simulink model "xts_system"  (R2026a)
settings: Solver=ode45  MaxStep=1e-2  AbsTol=1e-3
PreLoadFcn:
  | xts_PARAM
undefined symbols (not defined in the file or in its folder): sigbuilder_block, station_data, X, xts_rail_color, xts_rail_extr, xts_track_seg, Y, Z
libraries: sm_lib x28, xts_movers_lib x4, Multibody_Parts_Lib x4, nesl_utility x1
CloseFcn:
  | try,close(h1_xts_system),end
  | clear h1_xts_system
  | try,close(h2_xts_system),end
  | clear h2_xts_system
  | try,close(h3_xts_system),end
  | clear h3_xts_system
  | 
  | clear simlog_xts_system
  | clear logsout_xts_system
Description:
  | Linear Transport System
  | 
  | Copyright 2017-2026 The MathWorks, Inc.
settings Model: Creator=smiller  LastModifiedBy=smiller
settings DataIOCC: SignalLoggingName=logsout_xts_system
settings DebuggingCC: PregeneratedLibrarySubsystemCodeDiagnostic=none
settings SimscapeCC: SimscapeNormalizeSystem=off  SimscapeNominalValues="[{\"value\":\"1\",\"unit\":\"A\"},{\"value\":\"1\",\"unit\":\"bar\"},{\"value\":\"1\",\"unit\":\"cm^2\"},{\"value\":\"1\",\"unit\":\"cm^3/s\"},{\"value\":\"1\",\"unit\":\"kJ/kg\"},{\"value\":\"1\",\"unit\":\"kW\"},{\"value\":\"1\",\"unit\":\"l\"},{\"value\":\"1\",\"unit\":\"N\"},{\"value\":\"1\",\"unit\":\"N*m\"},{\"value\":\"1\",\"unit\":\"V\"}]"  SimscapeLogSimulationStatistics=on  SimscapeLogName=simlog_xts_system
settings DiagnosticsConfigSet: SimMechanicsUnconnectedFramePorts=none
settings ExplorerConfigSet: InternalSimMechanicsExplorerSettings="<ExplorerConfiguration><canonicalview>default</canonicalview><AnimationSetting><BasePlaybackSpeed>1.0</BasePlaybackSpeed><PlaybackSpeedFactor>1.0</PlaybackSpeedFactor></AnimationSetting><TilePanel><TileInfo><Tiles Columns=\"1\" Count=\"2\" Rows=\"2\"><Column Left=\"2\" Weight=\"1\"/><Column Left=\"429\"/><Row Top=\"2\" Weight=\"0.5743\"/><Row Top=\"165\" Weight=\"0.4257\"/><Row Top=\"287\"/><Tile Height=\"1\" Width=\"1\" X=\"0\" Y=\"0\"/><Tile Height=\"1\" Width=\"1\" X=\"0\" Y=\"1\"/></Tiles></TileInfo><SceneInfo><SceneViewer><BGColor><R>1</R><G>1</G><B>1</B></BGColor><Camera><DoPerspective>off</DoPerspective><Position><X>0.85235026960784244</X><Y>-0.74235025649298092</Y><Z>0.57735026635840536</Z></Position><Center><X>0.27500000041821659</X><Y>-0.16499998730335524</Y><Z>-2.831220369259313e-09</Z></Center><Up><X>-0.40824829046386307</X><Y>0.40824829046386307</Y><Z>0.81649658092772615</Z></Up><ViewLimDist>1</ViewLimDist><YLim>0.29785614758729934</YLim><XLim>0.80846668630838392</XLim></Camera></SceneViewer><SceneViewer><BGColor><R>1</R><G>1</G><B>1</B></BGColor><Camera><DoPerspective>on</DoPerspective><Position><X>-0.0044513318879480434</X><Y>-7.988545794836407e-05</Y><Z>0.039999999999999994</Z></Position><Center><X>0.99519221354671583</X><Y>0.026618093319754715</Y><Z>0.03999999999999955</Z></Center><Up><X>2.2204460492503131e-16</X><Y>0</Y><Z>0.99999999999999978</Z></Up><ViewLimDist>1</ViewLimDist><YLim>0.46630765815499858</YLim><XLim>1.7249256735291099</XLim></Camera></SceneViewer></SceneInfo></TilePanel><MechEditorPanel><Cameras><Camera><Id>Camera1</Id><Value><Name>Mover1</Name><NativeCamera><PositionTrackingFeature>Conveyor_1.Mover_1.Mover.Transform_Camera_1.F</PositionTrackingFeature><CenterTrackingFeature>Conveyor_1.Mover_1.Mover.Transform_Camera_1.F</CenterTrackingFeature><UpVectorTrackingFeature>Conveyor_1.Mover_1.Mover.Transform_Camera_1.F</UpVectorTrackingFeature><CenterTrackingOrigin>off</CenterTrackingOrigin><CenterTrackingDirection>-Z</CenterTrackingDirection><UpVectorTrackingDirection>-Y</UpVectorTrackingDirection></NativeCamera></Value></Camera></Cameras><GfxPanelCameraMap><MapElement CameraMLId=\"Camera1\" GfxPanelIndex=\"1\"/></GfxPanelCameraMap><VideoCreator><PlaybackSpeedRatio>1.0</PlaybackSpeedRatio><FrameRate>30</FrameRate><VideoFormat>Motion JPEG AVI</VideoFormat><FrameSize>auto</FrameSize></VideoCreator></MechEditorPanel></ExplorerConfiguration>"

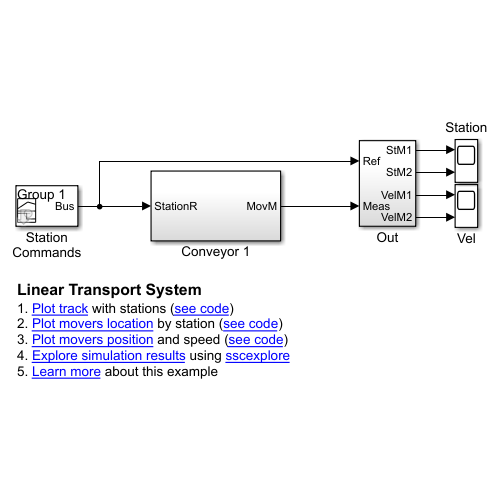
[thumbnail: Simulink's stored preview of the top-level diagram]
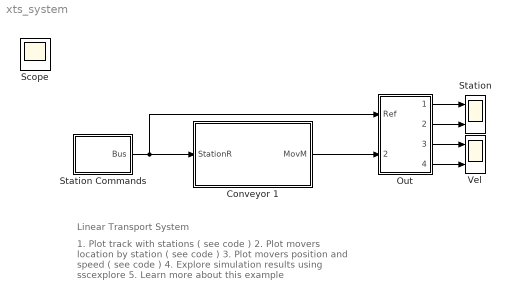
== system xts_system ==
  note: Linear Transport System
  note: 1. Plot track with stations ( see code )
      | 2. Plot movers location by station ( see code )
      | 3. Plot movers position and speed ( see code )
      | 4. Explore simulation results using sscexplore
      | 5. Learn more about this example
  Conveyor 1 : Subsystem  Tag=PublishSubsystem
  Out : Subsystem
  Station : Scope  NumInputPorts=2
      settings: ActiveDisplayYMinimum=-1.5  ActiveDisplayYMaximum=13.5  DataLoggingVariableName=ScopeData3
  Station Commands : Subsystem  Tag=STV Subsys  LoadFcn=sigbuilder_block('load');  StartFcn=sigbuilder_block('start');  StopFcn=sigbuilder_block('stop');  ClipboardFcn=sigbuilder_block('clipboard');  mask(Sigbuilder block){tuvar=[0:10]}
      mask help: Simulink:masks:SigbuilderBlock_MD
      mask init:
      | if ~strcmp(get_param(bdroot(gcbh),'SimulationStatus'),'stopped') tuvar = sigbuilder_block('maskInit'); end
      settings: CopyFcn=sigbuilder_block('copy');  DeleteFcn=sigbuilder_block('delete');  ModelCloseFcn=sigbuilder_block('modelClose');  PreSaveFcn=sigbuilder_block('preSave');  PauseFcn=sigbuilder_block('pause');  ContinueFcn=sigbuilder_block('continue');  NameChangeFcn=sigbuilder_block('namechange');  OpenFcn=sigbuilder_block('open',[437.6 199.2 550.4 400 ]);  CloseFcn=sigbuilder_block('close');
      mask Display: plot(0, 0, 100, 100,[2, 2, 32, 32, 2], [68, 8, 8, 68, 68],[32, 2], [38, 38], [32, 19, 2],[53, 60, 44], [32, 17, 17, 2],[16, 16, 31, 31]);txt = getActiveGroup(gcbh);text(2, 100, txt,'verticalAlignment', 'top');
  Vel : Scope  NumInputPorts=2
      settings: ActiveDisplayYMinimum=-0.12686  ActiveDisplayYMaximum=1.14176
  Scope : Scope
      settings: ActiveDisplayYMinimum=-6.25  ActiveDisplayYMaximum=56.25
  wires:
  Station Commands/1(Bus) -> Out/1(Ref), Conveyor 1/1(StationR)
  Conveyor 1/1(MovM) -> Out/2(Meas)
  Out/1(StM1) -> Station/1
  Out/2(StM2) -> Station/2
  Out/3(VelM1) -> Vel/1
  Out/4(VelM2) -> Vel/2

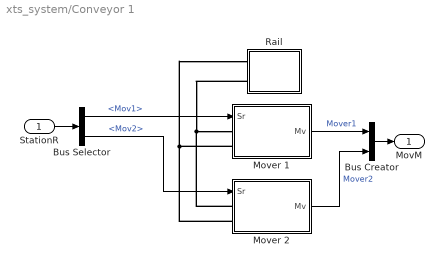
== system xts_system/Conveyor 1 ==
  StationR : Inport
  Bus Creator : BusCreator  Inputs=2
  Bus Selector : BusSelector  OutputSignals=Mov1,Mov2
  Mover 1 : Subsystem  Tag=PublishSubsystem
  Mover 2 : Subsystem
  Rail : Subsystem
  MovM : Outport  VectorParamsAs1DForOutWhenUnconnected=off
  wires:
  StationR/1 -> Bus Selector/1
  Bus Selector/1 -> Mover 1/1(Sr)  "<Mov1>"
  Bus Selector/2 -> Mover 2/1(Sr)  "<Mov2>"
  Mover 1/1(Mv) -> Bus Creator/1  "Mover1"
  Mover 2/1(Mv) -> Bus Creator/2  "Mover2"
  Bus Creator/1 -> MovM/1
  connections:
  Mover 1/LConn2 -- Mover 2/LConn2 -- Rail/RConn1
  Rail/RConn2 -- Mover 2/LConn1 -- Mover 1/LConn1

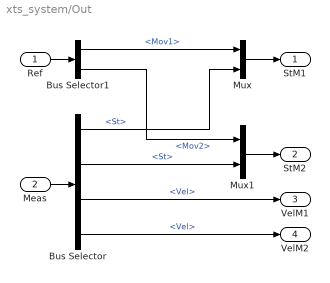
== system xts_system/Out ==
  Ref : Inport
  Meas : Inport  Port=2
  Bus Selector : BusSelector  OutputSignals=Mover1.St,Mover2.St,Mover1.Vel,Mover2.Vel
  Bus Selector1 : BusSelector  OutputSignals=Mov1,Mov2
  Mux : Mux  Inputs=2
  Mux1 : Mux  Inputs=2
  StM1 : Outport  VectorParamsAs1DForOutWhenUnconnected=off
  StM2 : Outport  Port=2  VectorParamsAs1DForOutWhenUnconnected=off
  VelM1 : Outport  Port=3  VectorParamsAs1DForOutWhenUnconnected=off
  VelM2 : Outport  Port=4  VectorParamsAs1DForOutWhenUnconnected=off
  wires:
  Bus Selector/1 -> Mux/2  "<St>"
  Mux/1 -> StM1/1
  Bus Selector1/2 -> Mux1/1  "<Mov2>"
  Mux1/1 -> StM2/1
  Bus Selector/4 -> VelM2/1  "<Vel>"
  Bus Selector/3 -> VelM1/1  "<Vel>"
  Bus Selector1/1 -> Mux/1  "<Mov1>"
  Meas/1 -> Bus Selector/1
  Bus Selector/2 -> Mux1/2  "<St>"
  Ref/1 -> Bus Selector1/1

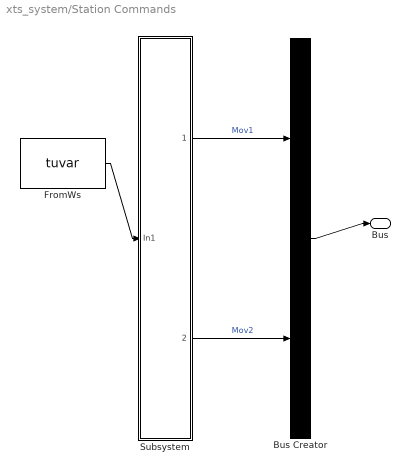
== system xts_system/Station Commands ==
  Bus Creator : BusCreator  Tag=Bus Creator  Inputs=2
  FromWs : FromWorkspace  Tag=STV FromWs  VariableName=tuvar
      SigBuilderData=|
      | common.afterFinalStr = 'Extrapolate'
      | common.sampleTime = 0
      | dataSet.timeRange = [0 10]
      | dataSet.name = 'Group 1'
      | sbobj.Groups.Name = 'Group 1'
      | sbobj.Groups.Signals(1).Name = 'Mov1'
      | sbobj.Groups.Signals(1).XData = [0 1.36 1.36 4 4 6 6 10]
      | sbobj.Groups.Signals(1).YData = [1 1 3 3 5 5 1 1]
      | sbobj.Groups.Signals(2).Name = 'Mov2'
      | sbobj.Groups.Signals(2).XData = [0 2.8 2.8 5 5 7.46 7.46 10]
      | sbobj.Groups.Signals(2).YData = [1 1 2 2 4 4 6 6]
  Subsystem : Subsystem
  Bus : Outport  VectorParamsAs1DForOutWhenUnconnected=off
  wires:
  FromWs/1 -> Subsystem/1(In1)
  Subsystem/1(Mov1) -> Bus Creator/1  "Mov1"
  Subsystem/2(Mov2) -> Bus Creator/2  "Mov2"
  Bus Creator/1 -> Bus/1

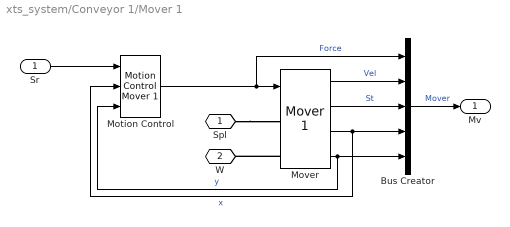
== system xts_system/Conveyor 1/Mover 1 ==
  Sr : Inport
  Bus Creator : BusCreator  Inputs=5
  Motion Control : xts_movers_lib/Motion Control Mover 1  dead_zone=xts_ctrl_dead_zone  max_force=xts_ctrl_max_force  err_gain_on_off=xts_ctrl_on_off_gain
  Mover : xts_movers_lib/Mover 1  Tag=PublishSubsystem  vis_popup=Native  visc_friction=xts_rail_visc_frict  init_pos_xy=[0 0]  station_data_o=station_o  station_data_x=station_x  station_data_y=station_y
  Spl : PMIOPort  Side=Left
  W : PMIOPort  Port=2  Side=Left
  Mv : Outport  VectorParamsAs1DForOutWhenUnconnected=off
  wires:
  Sr/1 -> Motion Control/1
  Mover/2 -> Bus Creator/3  "St"
  Mover/1 -> Bus Creator/2  "Vel"
  Motion Control/1 -> Bus Creator/1, Mover/1  "Force"
  Mover/3 -> Bus Creator/4, Motion Control/2  "x"
  Mover/4 -> Bus Creator/5, Motion Control/3  "y"
  Bus Creator/1 -> Mv/1  "Mover"
  connections:
  Mover/LConn2 -- W/RConn1
  Spl/RConn1 -- Mover/LConn1

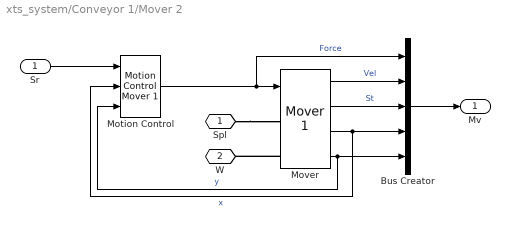
== system xts_system/Conveyor 1/Mover 2 ==
  Sr : Inport
  Bus Creator : BusCreator  Inputs=5
  Motion Control : xts_movers_lib/Motion Control Mover 1  dead_zone=xts_ctrl_dead_zone  max_force=xts_ctrl_max_force  err_gain_on_off=xts_ctrl_on_off_gain
  Mover : xts_movers_lib/Mover 1  vis_popup=Native  visc_friction=xts_rail_visc_frict  init_pos_xy=[0.5 0]  station_data_o=station_o  station_data_x=station_x  station_data_y=station_y
  Spl : PMIOPort  Side=Left
  W : PMIOPort  Port=2  Side=Left
  Mv : Outport  VectorParamsAs1DForOutWhenUnconnected=off
  wires:
  Bus Creator/1 -> Mv/1
  Mover/4 -> Motion Control/3, Bus Creator/5  "y"
  Mover/3 -> Motion Control/2, Bus Creator/4  "x"
  Motion Control/1 -> Mover/1, Bus Creator/1  "Force"
  Mover/1 -> Bus Creator/2  "Vel"
  Mover/2 -> Bus Creator/3  "St"
  Sr/1 -> Motion Control/1
  connections:
  Spl/RConn1 -- Mover/LConn1
  Mover/LConn2 -- W/RConn1

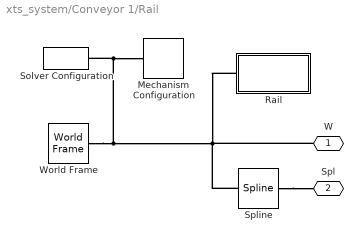
== system xts_system/Conveyor 1/Rail ==
  Mechanism Configuration : sm_lib/Utilities/Mechanism Configuration  UniformGravity=Constant  GravityVector=[0 -9.80665 0]*0  GravityVectorUnits=m/s^2  LinearizationDelta=0.001  JointModeTransitionNonlinearIterations=2
  Rail : Subsystem  Tag=PublishSubsystem  mask{rail_xc=xts_rail_extr, rail_seg=xts_track_seg, rail_color=xts_rail_color}
      mask prompts: rail_xc "Rail Cross-Section in x-y (m)"; rail_seg "Track Segments (len/rad, angle)"; rail_color "Rail Color (RGB)"
  Solver Configuration : nesl_utility/Solver Configuration  PhysicalDomain=network_engine_domain  SubClassName=solver  LeftPortType=input  RightPortType=generic  Tones=[]  Harmonics=[]  SimulateNoise=off  Profile=off  UseLocalSampling=off  EnableSwitchedLinearOptims=on  FrequencyDomain=off  UseCCode=off  RelTol=0.001  AbsTol=1e-06  MinStep=1e-09  ToWorkspace=off  RevertToSquareIcSolve=off  NumHomotopyIterations=100  PhasorMode=off  PhasorModeNumHarmonics=1  ConsistencySolver=NEWTON_FTOL  CanonicalOrdering=UNORDERED  OptimizeIntermediates=UNOPTIMIZED  IndexReductionMethod=DerivativeReplacement  DoDC=off  ResidualTolerance=1e-09  ConsistencyTolSource=GLOBAL  ConsistencyAbsTol=0.001  ConsistencyRelTol=0.001  ConsistencyTolFactor=0.001  UseLocalSolver=off  LocalSolverChoice=NE_BACKWARD_EULER_ADVANCER  ResolveIndetEquations=on  FunctionEvalNumThread=1  LocalSolverSampleTime=0.001  DoFixedCost=off  MaxNonlinIter=3  MaxModeIter=2  ComputeImpulses=off  ImpulseIterations=2  LinearAlgebra=Sparse  LinearAlgebraNumThread=0  EquationFormulation=NE_TIME_EF  DelaysMemoryBudget=1024  AutomaticFiltering=on  FilteringTimeConstant=0.001  PartitionStorageMethod=AS_NEEDED  PartitionMemoryBudget=1024  PartitionMethod=FAST  MultibodyUseLocalSolver=off  MultibodyLocalSolverChoice=ODE1  MultibodyLocalSolverSampleTime=0.001
  Spline : sm_lib/Curves and Surfaces/Spline  DataPoints=rail_spline  DataPointsUnits=m  EndConditionType=Closed  GraphicType=FromGeometry  MarkerShape=Sphere  MarkerSize=10  GraphicVisPropType=SimpleVisualProperties  GraphicDiffuseColor=[0 0 0]  GraphicOpacity=1.0  GraphicSpecularColor=[0.5 0.5 0.5 1.0]  GraphicAmbientColor=[0.15 0.15 0.15 1.0]  GraphicEmissiveColor=[0.0 0.0 0.0 1.0]  GraphicShininess=75
  World Frame : sm_lib/Frames and Transforms/World Frame
  W : PMIOPort  Side=Right
  Spl : PMIOPort  Port=2  Side=Right
  connections:
  Spline/RConn1 -- Spl/RConn1
  Solver Configuration/RConn1 -- W/RConn1 -- Spline/LConn1 -- Rail/LConn1 -- World Frame/RConn1 -- Mechanism Configuration/RConn1

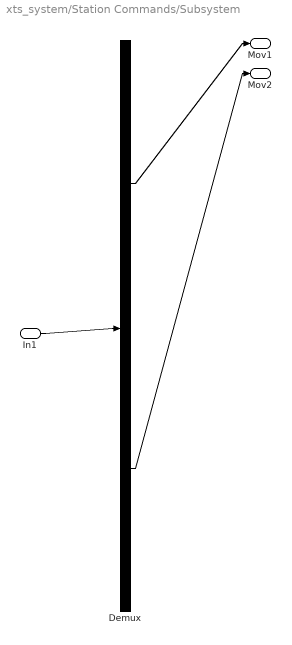
== system xts_system/Station Commands/Subsystem ==
  In1 : Inport
  Demux : Demux  Tag=STV Demux  Outputs=2
      settings: DisplayOption=none
  Mov1 : Outport  Tag=STV Outport  VectorParamsAs1DForOutWhenUnconnected=off
  Mov2 : Outport  Tag=STV Outport  Port=2  VectorParamsAs1DForOutWhenUnconnected=off
  wires:
  Demux/1 -> Mov1/1
  Demux/2 -> Mov2/1
  In1/1 -> Demux/1

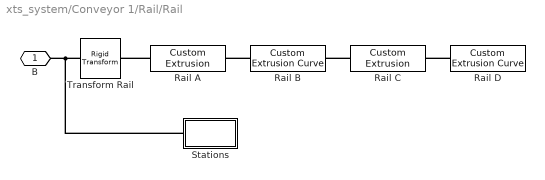
== system xts_system/Conveyor 1/Rail/Rail ==
  Rail A : Multibody_Parts_Lib/Extrusions/Custom Extrusion  extr_xsec=rail_xc  extr_len=rail_seg(1,1)  extr_rho=7000  extr_color=rail_color  extr_opc=1
      settings: SourceProductName=Simscape Multibody Parts Library
  Rail B : Multibody_Parts_Lib/Extrusions/Custom Extrusion Curve  extr_xsec=rail_xc  arc_rad=rail_seg(2,1)  arc_angle=rail_seg(2,2)  popup_arcdir=Y  extr_rho=7000  extr_color=rail_color  extr_opc=1
      settings: SourceProductName=Simscape Multibody Parts Library
  Rail C : Multibody_Parts_Lib/Extrusions/Custom Extrusion  extr_xsec=rail_xc  extr_len=rail_seg(3,1)  extr_rho=7000  extr_color=rail_color  extr_opc=1
      settings: SourceProductName=Simscape Multibody Parts Library
  Rail D : Multibody_Parts_Lib/Extrusions/Custom Extrusion Curve  extr_xsec=rail_xc  arc_rad=rail_seg(4,1)  arc_angle=rail_seg(4,2)  popup_arcdir=Y  extr_rho=7000  extr_color=rail_color  extr_opc=1
      settings: SourceProductName=Simscape Multibody Parts Library
  Stations : Subsystem
  Transform Rail : sm_lib/Frames and Transforms/Rigid Transform  RotationMethod=StandardAxis  FollAlignAxisA=+Z  BaseAlignAxisA=+X  FollAlignAxisB=+X  BaseAlignAxisB=-Y  RotationStandardAxis=+X  RotationAngle=-90  RotationAngleUnits=deg  RotationArbitraryAxis=[0 0 1]  RotationSequenceAxes=FollowerAxes  RotationSequence=XYX  RotationSequenceAngles=[0 0 0]  RotationSequenceAnglesUnits=deg  RotationMatrix=[1 0 0; 0 1 0; 0 0 1]  Quaternion=[1 0 0 0]  TranslationMethod=None  TranslationCartesianOffset=[0 0 0]  TranslationCartesianOffsetUnits=m  TranslationStandardAxis=+Z  TranslationStandardOffset=0  TranslationStandardOffsetUnits=m  TranslationROffset=0  TranslationROffsetUnits=m  TranslationThetaOffset=0  TranslationThetaOffsetUnits=deg  TranslationZOffset=0  TranslationZOffsetUnits=m
  B : PMIOPort  Side=Left
  connections:
  Stations/LConn1 -- Transform Rail/LConn1 -- B/RConn1
  Rail B/LConn1 -- Rail A/RConn1
  Rail D/LConn1 -- Rail C/RConn1
  Rail C/LConn1 -- Rail B/RConn1
  Rail A/LConn1 -- Transform Rail/RConn1

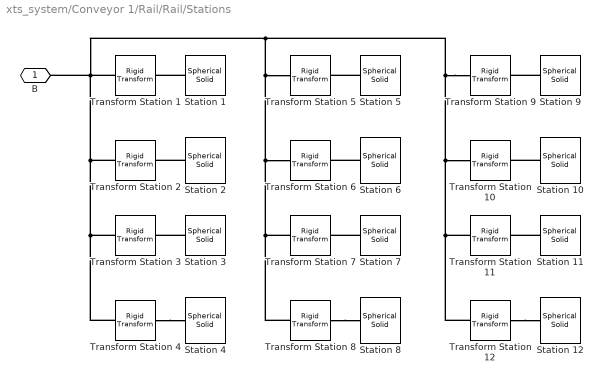
== system xts_system/Conveyor 1/Rail/Rail/Stations ==
  Station {1..12} (12 alike) : sm_lib/Body Elements/Spherical Solid  SphereRadius=0.05  SphereRadiusUnits=m  ExportEntireGeometry=off  InertiaType=CalculateFromGeometry  BasedOnType=Density  Density=1000  DensityUnits=kg/m^3  Mass=1  MassUnits=kg  CenterOfMass=[0 0 0]  CenterOfMassUnits=m  MomentsOfInertia=[1 1 1]  MomentsOfInertiaUnits=kg*m^2  ProductsOfInertia=[1 1 1]  ProductsOfInertiaUnits=kg*m^2  GraphicType=FromGeometry  MarkerShape=Sphere  MarkerSize=10  GraphicVisPropType=SimpleVisualProperties  GraphicDiffuseColor=[1.0 0.6 0.4]  GraphicOpacity=0.3  GraphicSpecularColor=[0.5 0.5 0.5 1.0]  GraphicAmbientColor=[0.15 0.15 0.15 1.0]  GraphicEmissiveColor=[0.0 0.0 0.0 1.0]  GraphicShininess=75  DoExposeReferenceFrame=on  SerializedFrames=<Frames/>
  Transform Station 1 : sm_lib/Frames and Transforms/Rigid Transform  RotationMethod=None  FollAlignAxisA=+X  BaseAlignAxisA=+Y  FollAlignAxisB=+Y  BaseAlignAxisB=+Z  RotationStandardAxis=+X  RotationAngle=0  RotationAngleUnits=deg  RotationArbitraryAxis=[0 0 1]  RotationSequenceAxes=FollowerAxes  RotationSequence=XYX  RotationSequenceAngles=[0 0 0]  RotationSequenceAnglesUnits=deg  RotationMatrix=[1 0 0; 0 1 0; 0 0 1]  Quaternion=[1 0 0 0]  TranslationMethod=Cartesian  TranslationCartesianOffset=[station_data(1,2) station_data(1,3) 0]  TranslationCartesianOffsetUnits=m  TranslationStandardAxis=+Z  TranslationStandardOffset=0  TranslationStandardOffsetUnits=m  TranslationROffset=0  TranslationROffsetUnits=m  TranslationThetaOffset=0  TranslationThetaOffsetUnits=deg  TranslationZOffset=0  TranslationZOffsetUnits=m
  Transform Station 10 : sm_lib/Frames and Transforms/Rigid Transform  RotationMethod=None  FollAlignAxisA=+X  BaseAlignAxisA=+Y  FollAlignAxisB=+Y  BaseAlignAxisB=+Z  RotationStandardAxis=+X  RotationAngle=0  RotationAngleUnits=deg  RotationArbitraryAxis=[0 0 1]  RotationSequenceAxes=FollowerAxes  RotationSequence=XYX  RotationSequenceAngles=[0 0 0]  RotationSequenceAnglesUnits=deg  RotationMatrix=[1 0 0; 0 1 0; 0 0 1]  Quaternion=[1 0 0 0]  TranslationMethod=Cartesian  TranslationCartesianOffset=[station_data(10,2) station_data(10,3) 0]  TranslationCartesianOffsetUnits=m  TranslationStandardAxis=+Z  TranslationStandardOffset=0  TranslationStandardOffsetUnits=m  TranslationROffset=0  TranslationROffsetUnits=m  TranslationThetaOffset=0  TranslationThetaOffsetUnits=deg  TranslationZOffset=0  TranslationZOffsetUnits=m
  Transform Station 11 : sm_lib/Frames and Transforms/Rigid Transform  RotationMethod=None  FollAlignAxisA=+X  BaseAlignAxisA=+Y  FollAlignAxisB=+Y  BaseAlignAxisB=+Z  RotationStandardAxis=+X  RotationAngle=0  RotationAngleUnits=deg  RotationArbitraryAxis=[0 0 1]  RotationSequenceAxes=FollowerAxes  RotationSequence=XYX  RotationSequenceAngles=[0 0 0]  RotationSequenceAnglesUnits=deg  RotationMatrix=[1 0 0; 0 1 0; 0 0 1]  Quaternion=[1 0 0 0]  TranslationMethod=Cartesian  TranslationCartesianOffset=[station_data(11,2) station_data(11,3) 0]  TranslationCartesianOffsetUnits=m  TranslationStandardAxis=+Z  TranslationStandardOffset=0  TranslationStandardOffsetUnits=m  TranslationROffset=0  TranslationROffsetUnits=m  TranslationThetaOffset=0  TranslationThetaOffsetUnits=deg  TranslationZOffset=0  TranslationZOffsetUnits=m
  Transform Station 12 : sm_lib/Frames and Transforms/Rigid Transform  RotationMethod=None  FollAlignAxisA=+X  BaseAlignAxisA=+Y  FollAlignAxisB=+Y  BaseAlignAxisB=+Z  RotationStandardAxis=+X  RotationAngle=0  RotationAngleUnits=deg  RotationArbitraryAxis=[0 0 1]  RotationSequenceAxes=FollowerAxes  RotationSequence=XYX  RotationSequenceAngles=[0 0 0]  RotationSequenceAnglesUnits=deg  RotationMatrix=[1 0 0; 0 1 0; 0 0 1]  Quaternion=[1 0 0 0]  TranslationMethod=Cartesian  TranslationCartesianOffset=[station_data(12,2) station_data(12,3) 0]  TranslationCartesianOffsetUnits=m  TranslationStandardAxis=+Z  TranslationStandardOffset=0  TranslationStandardOffsetUnits=m  TranslationROffset=0  TranslationROffsetUnits=m  TranslationThetaOffset=0  TranslationThetaOffsetUnits=deg  TranslationZOffset=0  TranslationZOffsetUnits=m
  Transform Station 2 : sm_lib/Frames and Transforms/Rigid Transform  RotationMethod=None  FollAlignAxisA=+X  BaseAlignAxisA=+Y  FollAlignAxisB=+Y  BaseAlignAxisB=+Z  RotationStandardAxis=+X  RotationAngle=0  RotationAngleUnits=deg  RotationArbitraryAxis=[0 0 1]  RotationSequenceAxes=FollowerAxes  RotationSequence=XYX  RotationSequenceAngles=[0 0 0]  RotationSequenceAnglesUnits=deg  RotationMatrix=[1 0 0; 0 1 0; 0 0 1]  Quaternion=[1 0 0 0]  TranslationMethod=Cartesian  TranslationCartesianOffset=[station_data(2,2) station_data(2,3) 0]  TranslationCartesianOffsetUnits=m  TranslationStandardAxis=+Z  TranslationStandardOffset=0  TranslationStandardOffsetUnits=m  TranslationROffset=0  TranslationROffsetUnits=m  TranslationThetaOffset=0  TranslationThetaOffsetUnits=deg  TranslationZOffset=0  TranslationZOffsetUnits=m
  Transform Station 3 : sm_lib/Frames and Transforms/Rigid Transform  RotationMethod=None  FollAlignAxisA=+X  BaseAlignAxisA=+Y  FollAlignAxisB=+Y  BaseAlignAxisB=+Z  RotationStandardAxis=+X  RotationAngle=0  RotationAngleUnits=deg  RotationArbitraryAxis=[0 0 1]  RotationSequenceAxes=FollowerAxes  RotationSequence=XYX  RotationSequenceAngles=[0 0 0]  RotationSequenceAnglesUnits=deg  RotationMatrix=[1 0 0; 0 1 0; 0 0 1]  Quaternion=[1 0 0 0]  TranslationMethod=Cartesian  TranslationCartesianOffset=[station_data(3,2) station_data(3,3) 0]  TranslationCartesianOffsetUnits=m  TranslationStandardAxis=+Z  TranslationStandardOffset=0  TranslationStandardOffsetUnits=m  TranslationROffset=0  TranslationROffsetUnits=m  TranslationThetaOffset=0  TranslationThetaOffsetUnits=deg  TranslationZOffset=0  TranslationZOffsetUnits=m
  Transform Station 4 : sm_lib/Frames and Transforms/Rigid Transform  RotationMethod=None  FollAlignAxisA=+X  BaseAlignAxisA=+Y  FollAlignAxisB=+Y  BaseAlignAxisB=+Z  RotationStandardAxis=+X  RotationAngle=0  RotationAngleUnits=deg  RotationArbitraryAxis=[0 0 1]  RotationSequenceAxes=FollowerAxes  RotationSequence=XYX  RotationSequenceAngles=[0 0 0]  RotationSequenceAnglesUnits=deg  RotationMatrix=[1 0 0; 0 1 0; 0 0 1]  Quaternion=[1 0 0 0]  TranslationMethod=Cartesian  TranslationCartesianOffset=[station_data(4,2) station_data(4,3) 0]  TranslationCartesianOffsetUnits=m  TranslationStandardAxis=+Z  TranslationStandardOffset=0  TranslationStandardOffsetUnits=m  TranslationROffset=0  TranslationROffsetUnits=m  TranslationThetaOffset=0  TranslationThetaOffsetUnits=deg  TranslationZOffset=0  TranslationZOffsetUnits=m
  Transform Station 5 : sm_lib/Frames and Transforms/Rigid Transform  RotationMethod=None  FollAlignAxisA=+X  BaseAlignAxisA=+Y  FollAlignAxisB=+Y  BaseAlignAxisB=+Z  RotationStandardAxis=+X  RotationAngle=0  RotationAngleUnits=deg  RotationArbitraryAxis=[0 0 1]  RotationSequenceAxes=FollowerAxes  RotationSequence=XYX  RotationSequenceAngles=[0 0 0]  RotationSequenceAnglesUnits=deg  RotationMatrix=[1 0 0; 0 1 0; 0 0 1]  Quaternion=[1 0 0 0]  TranslationMethod=Cartesian  TranslationCartesianOffset=[station_data(5,2) station_data(5,3) 0]  TranslationCartesianOffsetUnits=m  TranslationStandardAxis=+Z  TranslationStandardOffset=0  TranslationStandardOffsetUnits=m  TranslationROffset=0  TranslationROffsetUnits=m  TranslationThetaOffset=0  TranslationThetaOffsetUnits=deg  TranslationZOffset=0  TranslationZOffsetUnits=m
  Transform Station 6 : sm_lib/Frames and Transforms/Rigid Transform  RotationMethod=None  FollAlignAxisA=+X  BaseAlignAxisA=+Y  FollAlignAxisB=+Y  BaseAlignAxisB=+Z  RotationStandardAxis=+X  RotationAngle=0  RotationAngleUnits=deg  RotationArbitraryAxis=[0 0 1]  RotationSequenceAxes=FollowerAxes  RotationSequence=XYX  RotationSequenceAngles=[0 0 0]  RotationSequenceAnglesUnits=deg  RotationMatrix=[1 0 0; 0 1 0; 0 0 1]  Quaternion=[1 0 0 0]  TranslationMethod=Cartesian  TranslationCartesianOffset=[station_data(6,2) station_data(6,3) 0]  TranslationCartesianOffsetUnits=m  TranslationStandardAxis=+Z  TranslationStandardOffset=0  TranslationStandardOffsetUnits=m  TranslationROffset=0  TranslationROffsetUnits=m  TranslationThetaOffset=0  TranslationThetaOffsetUnits=deg  TranslationZOffset=0  TranslationZOffsetUnits=m
  Transform Station 7 : sm_lib/Frames and Transforms/Rigid Transform  RotationMethod=None  FollAlignAxisA=+X  BaseAlignAxisA=+Y  FollAlignAxisB=+Y  BaseAlignAxisB=+Z  RotationStandardAxis=+X  RotationAngle=0  RotationAngleUnits=deg  RotationArbitraryAxis=[0 0 1]  RotationSequenceAxes=FollowerAxes  RotationSequence=XYX  RotationSequenceAngles=[0 0 0]  RotationSequenceAnglesUnits=deg  RotationMatrix=[1 0 0; 0 1 0; 0 0 1]  Quaternion=[1 0 0 0]  TranslationMethod=Cartesian  TranslationCartesianOffset=[station_data(7,2) station_data(7,3) 0]  TranslationCartesianOffsetUnits=m  TranslationStandardAxis=+Z  TranslationStandardOffset=0  TranslationStandardOffsetUnits=m  TranslationROffset=0  TranslationROffsetUnits=m  TranslationThetaOffset=0  TranslationThetaOffsetUnits=deg  TranslationZOffset=0  TranslationZOffsetUnits=m
  Transform Station 8 : sm_lib/Frames and Transforms/Rigid Transform  RotationMethod=None  FollAlignAxisA=+X  BaseAlignAxisA=+Y  FollAlignAxisB=+Y  BaseAlignAxisB=+Z  RotationStandardAxis=+X  RotationAngle=0  RotationAngleUnits=deg  RotationArbitraryAxis=[0 0 1]  RotationSequenceAxes=FollowerAxes  RotationSequence=XYX  RotationSequenceAngles=[0 0 0]  RotationSequenceAnglesUnits=deg  RotationMatrix=[1 0 0; 0 1 0; 0 0 1]  Quaternion=[1 0 0 0]  TranslationMethod=Cartesian  TranslationCartesianOffset=[station_data(8,2) station_data(8,3) 0]  TranslationCartesianOffsetUnits=m  TranslationStandardAxis=+Z  TranslationStandardOffset=0  TranslationStandardOffsetUnits=m  TranslationROffset=0  TranslationROffsetUnits=m  TranslationThetaOffset=0  TranslationThetaOffsetUnits=deg  TranslationZOffset=0  TranslationZOffsetUnits=m
  Transform Station 9 : sm_lib/Frames and Transforms/Rigid Transform  RotationMethod=None  FollAlignAxisA=+X  BaseAlignAxisA=+Y  FollAlignAxisB=+Y  BaseAlignAxisB=+Z  RotationStandardAxis=+X  RotationAngle=0  RotationAngleUnits=deg  RotationArbitraryAxis=[0 0 1]  RotationSequenceAxes=FollowerAxes  RotationSequence=XYX  RotationSequenceAngles=[0 0 0]  RotationSequenceAnglesUnits=deg  RotationMatrix=[1 0 0; 0 1 0; 0 0 1]  Quaternion=[1 0 0 0]  TranslationMethod=Cartesian  TranslationCartesianOffset=[station_data(9,2) station_data(9,3) 0]  TranslationCartesianOffsetUnits=m  TranslationStandardAxis=+Z  TranslationStandardOffset=0  TranslationStandardOffsetUnits=m  TranslationROffset=0  TranslationROffsetUnits=m  TranslationThetaOffset=0  TranslationThetaOffsetUnits=deg  TranslationZOffset=0  TranslationZOffsetUnits=m
  B : PMIOPort  Side=Left
  connections:
  Station 1/RConn1 -- Transform Station 1/RConn1
  Transform Station 9/LConn1 -- Transform Station 7/LConn1 -- Transform Station 8/LConn1 -- Transform Station 6/LConn1 -- Transform Station 5/LConn1 -- Transform Station 4/LConn1 -- Transform Station 3/LConn1 -- Transform Station 2/LConn1 -- B/RConn1 -- Transform Station 1/LConn1 -- Transform Station 10/LConn1 -- Transform Station 12/LConn1 -- Transform Station 11/LConn1
  Station 2/RConn1 -- Transform Station 2/RConn1
  Station 3/RConn1 -- Transform Station 3/RConn1
  Transform Station 4/RConn1 -- Station 4/RConn1
  Station 6/RConn1 -- Transform Station 6/RConn1
  Station 7/RConn1 -- Transform Station 7/RConn1
  Transform Station 8/RConn1 -- Station 8/RConn1
  Station 5/RConn1 -- Transform Station 5/RConn1
  Station 9/RConn1 -- Transform Station 9/RConn1
  Transform Station 12/RConn1 -- Station 12/RConn1
  Station 11/RConn1 -- Transform Station 11/RConn1
  Station 10/RConn1 -- Transform Station 10/RConn1
